simulink library "lib_filtered_derivative"  (R2023a)
settings: Solver=VariableStepAuto  StartTime=0.0  StopTime=10.0  RelTol=1e-3
undefined symbols (not defined in the file): parElctSpdMaxVal, parMedTaskSampTime_u16d6b0
libraries: lib_conversion x10, lib_resettable_unit_delay x2, lib_configurable_parameter x2
settings Model: Creator=cav2ofo  LastModifiedBy=lenovo
settings OptimizationCC: ReuseModelBlockBuffer=off

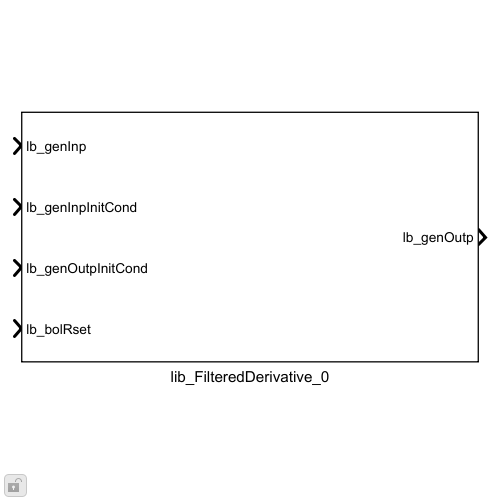
[thumbnail: Simulink's stored preview of the top-level diagram]
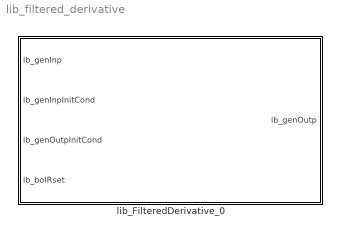
== system lib_filtered_derivative ==
  lib_FilteredDerivative_0 : Subsystem  mask{lb_parSampTime=parMedTaskSampTime_u16d6b0, lb_parTimeCnst=1e-3, lb_parMaxTimeCnst=1e-1, lb_parMinTimeCnst=1e-4, lb_parMaxOutpVal=parElctSpdMaxVal, lb_parAngInpMode=on, lb_parIIntrDataTypeMode=32-bit, lb_parOutpDataType=fixdt(1,16,2^-3,0)}
      mask prompts: lb_parSampTime "Sampling time [s]:"; lb_parTimeCnst "Time constant [s]:"; lb_parMaxTimeCnst "Maximum time constant [s]:"; lb_parMinTimeCnst "Minimum time constant [s]:"; lb_parMaxOutpVal "Maximum output value [ou]:"; lb_parAngInpMode "Angle input mode"; lb_parIIntrDataTypeMode "Internal data types mode:"; lb_parOutpDataType "Output data type:"
      mask init:
      | %% Determine number of bits for internal data types
      | switch lb_parIIntrDataTypeMode
      |     case 'Same of output'
      |         temp.bitNum_scl = lb_parOutpDataType.WordLength;
      |     case '32-bit'
      |         temp.bitNum_scl = 32;
      | end
      | 
      | %% Compute data type for parameter cnst1=Ts+Tc
      | lb_parCnst1MaxVal = double(lb_parSampTime)+lb_parMaxTimeCnst;
      | lb_parCnst1DataType = Simulink.NumericType;
      | lb_parCnst1DataType.DataTypeMode = 'Fixed-point: unspecified scaling';
      | lb_parCnst1DataType.Signedness = 'Unsigned';
      | lb_parCnst1DataType.WordLength = 16;
      | 
      | %% Compute data type for parameter cnst2=Tc/(Ts+Tc)
      | lb_parCnst2MaxVal = lb_parMaxTimeCnst/(double(lb_parSampTime)+lb_parMinTimeCnst);
      | lb_parCnst2DataType = Simulink.NumericType;
      | lb_parCnst2DataType.DataTypeMode = 'Fixed-point: unspecified scaling';
      | lb_parCnst2DataType.Signedness = 'Unsigned';
      | lb_parCnst2DataType.WordLength = 16;
      | 
      | %% Compute data type for parameter cnst3=1/(Ts+Tc)
      | lb_parCnst3MaxVal = 1/(double(lb_parSampTime)+lb_parMinTimeCnst);
      | lb_parCnst3DataType = Simulink.NumericType;
      | lb_parCnst3DataType.DataTypeMode = 'Fixed-point: unspecified scaling';
      | lb_parCnst3DataType.Signedness = 'Unsigned';
      | lb_parCnst3DataType.WordLength = 16;
      | 
      | %% Compute data type for feedfoward term of output
      | lb_parFdfwTermMaxVal = (lb_parMaxOutpVal*double(lb_parSampTime))/(double(lb_parSampTime)+lb_parMinTimeCnst);
      | lb_parFdfwTermDataType = Simulink.NumericType;
      | lb_parFdfwTermDataType.DataTypeMode = 'Fixed-point: unspecified scaling';
      | lb_parFdfwTermDataType.Signedness = 'Signed';
      | lb_parFdfwTermDataType.WordLength = temp.bitNum_scl;
      | 
      | %% Compute data type for feedback term of output
      | lb_parFdbkTermMaxVal = lb_parMaxOutpVal*lb_parCnst2MaxVal;
      | lb_parFdbkTermDataType = Simulink.NumericType;
      | lb_parFdbkTermDataType.DataTypeMode = 'Fixed-point: unspecified scaling';
      | lb_parFdbkTermDataType.Signedness = 'Signed';
      | lb_parFdbkTermDataType.WordLength = temp.bitNum_scl;
      | 
      | %% Compute data type for feedbacked output
      | lb_parAccmDataTypeMaxVal =  lb_parFdfwTermMaxVal+lb_parFdbkTermMaxVal;
      | lb_parAccmDataType = Simulink.NumericType;
      | lb_parAccmDataType.DataTypeMode = 'Fixed-point: unspecified scaling';
      | lb_parAccmDataType.Signedness = 'Signed';
      | lb_parAccmDataType.WordLength = temp.bitNum_scl;
      | 
      | %% Assign common properties for data type used for input variation
      | lb_parInpVrtnDataType = Simulink.NumericType;
      | lb_parInpVrtnDataType.DataTypeMode = 'Fixed-point: slope and bias scaling';
      | lb_parInpVrtnDataType.Signedness = 'Signed';
      | lb_parInpVrtnDataType.WordLength = temp.bitNum_scl;
      | 
      | switch lb_parAngInpMode
      |     case 'on'
      |         
      |         %% Specify slope for input variation data type
      |         if lb_parInpVrtnDataType.WordLength == 32
      |             lb_parInpVrtnDataType.Slope = pi*2^-31;
      |         else
      |             lb_parInpVrtnDataType.Slope = pi*2^-15;
      |         end
      |         
      |         %% Activate angle mode variant
      |         set_param([gcb,'/sss_InputVariationComputation/vss_InputMode'],...
      |             'LabelModeActiveChoice','lb_parAngInpModeLbl');
      |     case 'off'
      |         
      |         %% Specify slope for input variation data type
      |         temp.DataType_obj = fi(lb_parMaxOutpVal*double(lb_parSampTime),1,temp.bitNum_scl);
      |         lb_parInpVrtnDataType.Slope = 2^-temp.DataType_obj.FractionLength;
      |         
      |         %% Deactivate angle mode variant
      |         set_param([gcb,'/sss_InputVariationComputation/vss_InputMode'],...
      |             'LabelModeActiveChoice','lb_parNoAngInpModeLbl');
      | end
      | 
      | clear temp;
      mask TypeOptions lb_parIIntrDataTypeMode: Same of output | 32-bit
      mask DialogControl DescGroupVar Prompt: VHIT control library
      mask DialogControl DescTextVar Prompt: Filtered derivative
      mask DialogControl Container3 Prompt: Data type

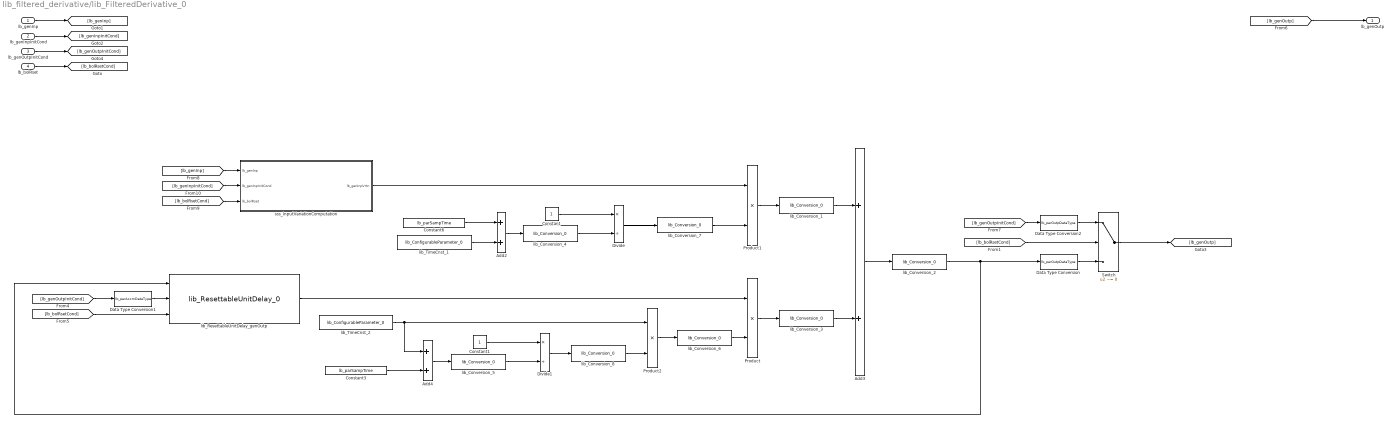
== system lib_filtered_derivative/lib_FilteredDerivative_0 ==
  lb_genInp : Inport
  lb_genInpInitCond : Inport  Port=2
  lb_genOutpInitCond : Inport  Port=3
  lb_bolRset : Inport  Port=4
  Add2 : Sum  OutDataTypeStr=Inherit: Inherit via back propagation  RndMeth=Simplest
  Add3 : Sum  OutDataTypeStr=Inherit: Inherit via back propagation  RndMeth=Simplest
  Add4 : Sum  OutDataTypeStr=Inherit: Inherit via back propagation  RndMeth=Simplest
  Constant : Constant  OutDataTypeStr=fixdt(0,16,2^-15,0)
  Constant1 : Constant  OutDataTypeStr=fixdt(0,16,2^-15,0)
  Constant3 : Constant  Value=lb_parSampTime
  Constant6 : Constant  Value=lb_parSampTime
  Data Type Conversion : DataTypeConversion  OutDataTypeStr=lb_parOutpDataType  SaturateOnIntegerOverflow=off  RndMeth=Floor
  Data Type Conversion1 : DataTypeConversion  OutMax=lb_parAccmDataTypeMaxVal  OutDataTypeStr=lb_parAccmDataType  SaturateOnIntegerOverflow=off  RndMeth=Floor
  Data Type Conversion2 : DataTypeConversion  OutDataTypeStr=lb_parOutpDataType  SaturateOnIntegerOverflow=off  RndMeth=Floor
  Divide : Product  Inputs=*/  OutDataTypeStr=Inherit: Inherit via back propagation  RndMeth=Simplest
  Divide1 : Product  Inputs=*/  OutDataTypeStr=Inherit: Inherit via back propagation  RndMeth=Simplest
  Product : Product  OutDataTypeStr=Inherit: Inherit via back propagation  RndMeth=Simplest
  Product1 : Product  OutDataTypeStr=Inherit: Inherit via back propagation  RndMeth=Simplest
  Product2 : Product  OutDataTypeStr=Inherit: Inherit via back propagation  RndMeth=Simplest
  Switch : Switch  Criteria=u2 ~= 0  SaturateOnIntegerOverflow=off  InputSameDT=off
  lib_Conversion_1 : lib_conversion/lib_Conversion_0  lb_parDataType=lb_parFdfwTermDataType  lb_parOutpMaxVal=lb_parFdfwTermMaxVal  lb_parOutpMinVal=[]  RndMeth=Simplest  lb_parSatFlag=off
  lib_Conversion_2 : lib_conversion/lib_Conversion_0  lb_parDataType=lb_parAccmDataType  lb_parOutpMaxVal=lb_parAccmDataTypeMaxVal  lb_parOutpMinVal=[]  RndMeth=Simplest  lb_parSatFlag=off
  lib_Conversion_3 : lib_conversion/lib_Conversion_0  lb_parDataType=lb_parFdbkTermDataType  lb_parOutpMaxVal=lb_parFdbkTermMaxVal  lb_parOutpMinVal=[]  RndMeth=Simplest  lb_parSatFlag=off
  lib_Conversion_4 : lib_conversion/lib_Conversion_0  lb_parDataType=lb_parCnst1DataType  lb_parOutpMaxVal=lb_parCnst1MaxVal  lb_parOutpMinVal=[]  RndMeth=Simplest  lb_parSatFlag=off
  lib_Conversion_5 : lib_conversion/lib_Conversion_0  lb_parDataType=lb_parCnst1DataType  lb_parOutpMaxVal=lb_parCnst1MaxVal  lb_parOutpMinVal=[]  RndMeth=Simplest  lb_parSatFlag=off
  lib_Conversion_6 : lib_conversion/lib_Conversion_0  lb_parDataType=lb_parCnst2DataType  lb_parOutpMaxVal=lb_parCnst2MaxVal  lb_parOutpMinVal=[]  RndMeth=Simplest  lb_parSatFlag=off
  lib_Conversion_7 : lib_conversion/lib_Conversion_0  lb_parDataType=lb_parCnst3DataType  lb_parOutpMaxVal=lb_parCnst3MaxVal  lb_parOutpMinVal=[]  RndMeth=Simplest  lb_parSatFlag=off
  lib_Conversion_8 : lib_conversion/lib_Conversion_0  lb_parDataType=lb_parCnst3DataType  lb_parOutpMaxVal=lb_parCnst3MaxVal  lb_parOutpMinVal=[]  RndMeth=Simplest  lb_parSatFlag=off
  lib_ResettableUnitDelay_genOutp : lib_resettable_unit_delay/lib_ResettableUnitDelay_0
  lib_TimeCnst_1 : lib_configurable_parameter/lib_ConfigurableParameter_0  lb_parCnfgPar=lb_parTimeCnst  lb_parDataType=Inherit: Inherit from 'Constant value'  lb_parUpLim=lb_parMaxTimeCnst  lb_parLowLim=lb_parMinTimeCnst
  lib_TimeCnst_2 : lib_configurable_parameter/lib_ConfigurableParameter_0  lb_parCnfgPar=lb_parTimeCnst  lb_parDataType=Inherit: Inherit from 'Constant value'  lb_parUpLim=lb_parMaxTimeCnst  lb_parLowLim=lb_parMinTimeCnst
  sss_InputVariationComputation : Subsystem
  lb_genOutp : Outport
  wires:
  Constant3/1 -> Add4/2
  lib_Conversion_6/1 -> Product/2
  Product2/1 -> lib_Conversion_6/1
  lib_TimeCnst_2/1 -> Product2/1, Add4/1
  lb_genInpInitCond/1 -> [lb_genInpInitCond]
  lb_genInp/1 -> [lb_genInp]
  lb_genOutpInitCond/1 -> [lb_genOutpInitCond]
  lb_bolRset/1 -> [lb_bolRsetCond]
  [lb_bolRsetCond] -> lib_ResettableUnitDelay_genOutp/3
  lib_ResettableUnitDelay_genOutp/1 -> Product/1
  Product/1 -> lib_Conversion_3/1
  Product1/1 -> lib_Conversion_1/1
  Add3/1 -> lib_Conversion_2/1
  Constant6/1 -> Add2/1
  lib_TimeCnst_1/1 -> Add2/2
  [lb_genOutp] -> lb_genOutp/1
  Add4/1 -> lib_Conversion_5/1
  Add2/1 -> lib_Conversion_4/1
  lib_Conversion_4/1 -> Divide/2
  [lb_genInp] -> sss_InputVariationComputation/1(lb_genInp)
  [lb_bolRsetCond] -> sss_InputVariationComputation/3(lb_bolRset)
  [lb_genInpInitCond] -> sss_InputVariationComputation/2(lb_genInpInitCond)
  lib_Conversion_1/1 -> Add3/1
  lib_Conversion_3/1 -> Add3/2
  [lb_genOutpInitCond] -> Data Type Conversion1/1
  Data Type Conversion1/1 -> lib_ResettableUnitDelay_genOutp/2
  [lb_bolRsetCond] -> Switch/2
  lib_Conversion_2/1 -> Data Type Conversion/1, lib_ResettableUnitDelay_genOutp/1
  Switch/1 -> [lb_genOutp]
  [lb_genOutpInitCond] -> Data Type Conversion2/1
  Data Type Conversion2/1 -> Switch/1
  Data Type Conversion/1 -> Switch/3
  sss_InputVariationComputation/1(lb_genInpVrtn) -> Product1/1
  Constant/1 -> Divide/1
  Divide/1 -> lib_Conversion_7/1
  Constant1/1 -> Divide1/1
  lib_Conversion_5/1 -> Divide1/2
  Divide1/1 -> lib_Conversion_8/1
  lib_Conversion_7/1 -> Product1/2
  lib_Conversion_8/1 -> Product2/2

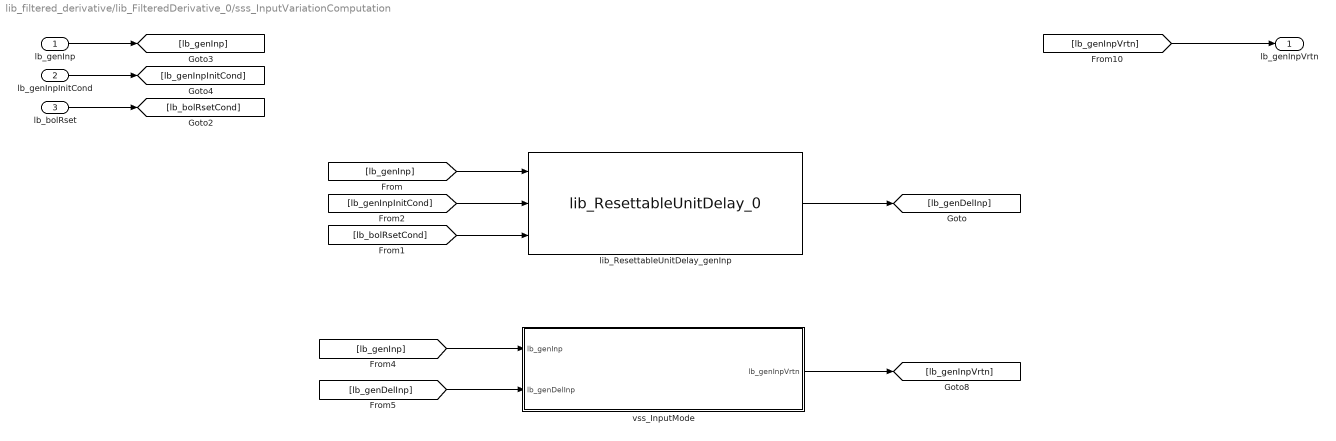
== system lib_filtered_derivative/lib_FilteredDerivative_0/sss_InputVariationComputation ==
  lb_genInp : Inport
  lb_genInpInitCond : Inport  Port=2
  lb_bolRset : Inport  Port=3
  lib_ResettableUnitDelay_genInp : lib_resettable_unit_delay/lib_ResettableUnitDelay_0
      settings: LibrarySourceBlock=vhit_control_library/lib_ResettableUnitDelay_0
  vss_InputMode : Subsystem  Variant=on  VariantControlMode=label  LabelModeActiveChoice=lb_parAngInpModeLbl
  lb_genInpVrtn : Outport
  wires:
  lb_bolRset/1 -> [lb_bolRsetCond]
  lb_genInp/1 -> [lb_genInp]
  lb_genInpInitCond/1 -> [lb_genInpInitCond]
  lib_ResettableUnitDelay_genInp/1 -> [lb_genDelInp]
  [lb_genInpInitCond] -> lib_ResettableUnitDelay_genInp/2
  [lb_bolRsetCond] -> lib_ResettableUnitDelay_genInp/3
  [lb_genInp] -> lib_ResettableUnitDelay_genInp/1
  vss_InputMode/1(lb_genInpVrtn) -> [lb_genInpVrtn]
  [lb_genInpVrtn] -> lb_genInpVrtn/1
  [lb_genDelInp] -> vss_InputMode/2(lb_genDelInp)
  [lb_genInp] -> vss_InputMode/1(lb_genInp)

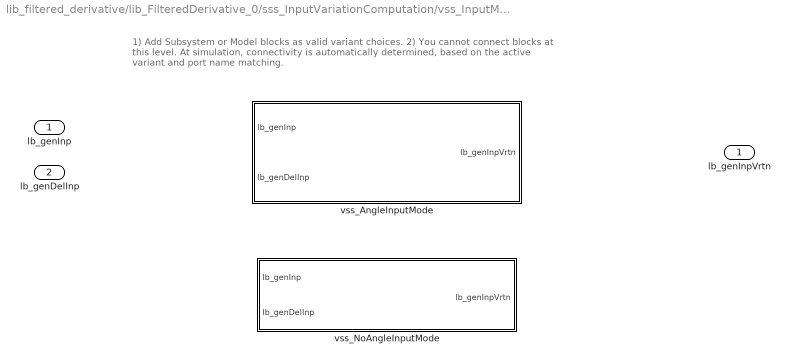
== system lib_filtered_derivative/lib_FilteredDerivative_0/sss_InputVariationComputation/vss_InputMode ==
  note: 1) Add Subsystem or Model blocks as valid variant choices.
      | 2) You cannot connect blocks at this level. At simulation, connectivity is automatically
      | determined, based on the active variant and port name matching.
  lb_genInp : Inport
  lb_genDelInp : Inport  Port=2
  vss_AngleInputMode : Subsystem  VariantControl=lb_parAngInpModeLbl
  vss_NoAngleInputMode : Subsystem  VariantControl=lb_parNoAngInpModeLbl
  lb_genInpVrtn : Outport

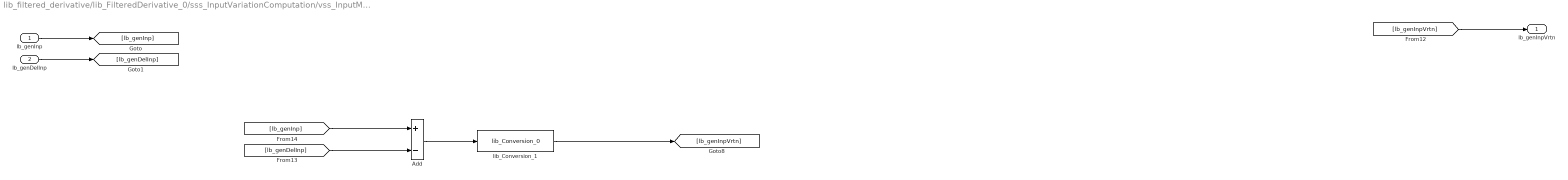
== system lib_filtered_derivative/lib_FilteredDerivative_0/sss_InputVariationComputation/vss_InputMode/vss_AngleInputMode ==
  lb_genInp : Inport
  lb_genDelInp : Inport  Port=2
  Add : Sum  Inputs=+-  OutDataTypeStr=Inherit: Inherit via back propagation  RndMeth=Simplest
  lib_Conversion_1 : lib_conversion/lib_Conversion_0  lb_parDataType=lb_parInpVrtnDataType  lb_parOutpMaxVal=[]  lb_parOutpMinVal=[]  lb_parSatFlag=off
  lb_genInpVrtn : Outport
  wires:
  lib_Conversion_1/1 -> [lb_genInpVrtn]
  [lb_genInpVrtn] -> lb_genInpVrtn/1
  lb_genDelInp/1 -> [lb_genDelInp]
  lb_genInp/1 -> [lb_genInp]
  Add/1 -> lib_Conversion_1/1
  [lb_genInp] -> Add/1
  [lb_genDelInp] -> Add/2

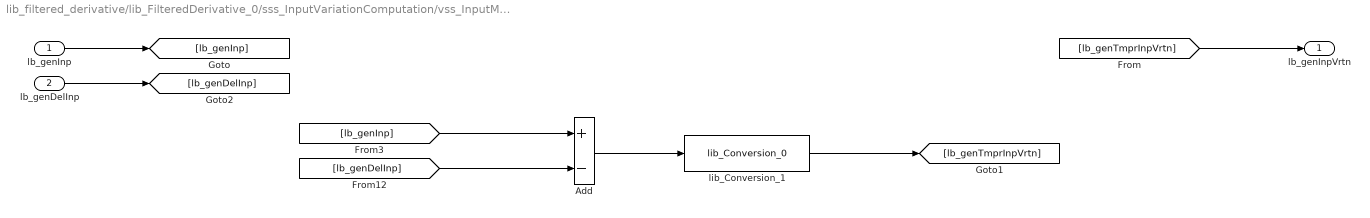
== system lib_filtered_derivative/lib_FilteredDerivative_0/sss_InputVariationComputation/vss_InputMode/vss_NoAngleInputMode ==
  lb_genInp : Inport
  lb_genDelInp : Inport  Port=2
  Add : Sum  Inputs=+-  OutDataTypeStr=Inherit: Inherit via back propagation  RndMeth=Simplest
  lib_Conversion_1 : lib_conversion/lib_Conversion_0  lb_parDataType=lb_parInpVrtnDataType  lb_parOutpMaxVal=[]  lb_parOutpMinVal=[]  lb_parSatFlag=off
  lb_genInpVrtn : Outport
  wires:
  [lb_genTmprInpVrtn] -> lb_genInpVrtn/1
  Add/1 -> lib_Conversion_1/1
  [lb_genInp] -> Add/1
  [lb_genDelInp] -> Add/2
  lib_Conversion_1/1 -> [lb_genTmprInpVrtn]
  lb_genDelInp/1 -> [lb_genDelInp]
  lb_genInp/1 -> [lb_genInp]
